simulink model "write_data_2018a"  (R2018a)
settings: Solver=FixedStepAuto  StartTime=0.0  StopTime=0.0001  RelTol=1e-3
values from neighbouring files (symbols this model uses):
  transfer_array = zeros(1,30)    [final_test.m]    (also in main_file.m = calc_corr_arr(transfer_array, v_m))
libraries: TcAdsLib x3
settings Model: Creator=chijiang  LastModifiedBy=chduan
settings OptimizationCC: LocalBlockOutputs=off
settings SFSimCC: SimUseLocalCustomCode=on
settings RTWCC: SystemTargetFile=TwinCAT.tlc  MakeCommand=make_tct  TemplateMakefile=tct_msbuild.tmf  Description=TwinCAT Target  GenerateReport=on  RTWUseLocalCustomCode=on  TargetLang=C++
settings STFCustomTargetCC: TargetLangStandard=C++03 (ISO)  CompOptLevelCompliant=on  MATLABClassNameForMDSCustomization=Simulink.SoftwareTarget.TargetSpecificTriggerConfigurationBase  SystemTargetFile=TwinCAT.tlc

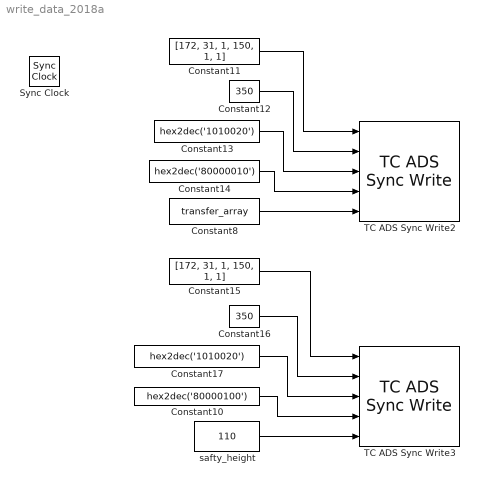
== system write_data_2018a ==
  Constant10 : Constant  Value=hex2dec('80000100')  OutDataTypeStr=uint32
  Constant11 : Constant  Value=[172, 31, 1, 150, 1, 1]  OutDataTypeStr=uint8
  Constant12 : Constant  Value=350  OutDataTypeStr=uint16
  Constant13 : Constant  Value=hex2dec('1010020')  OutDataTypeStr=uint32
  Constant14 : Constant  Value=hex2dec('80000010')  OutDataTypeStr=uint32
  Constant15 : Constant  Value=[172, 31, 1, 150, 1, 1]  OutDataTypeStr=uint8
  Constant16 : Constant  Value=350  OutDataTypeStr=uint16
  Constant17 : Constant  Value=hex2dec('1010020')  OutDataTypeStr=uint32
  Constant8 : Constant  Value=transfer_array
  Sync Clock : TcAdsLib/Utilities/Sync Clock  OutputPortSelect=None  InputPortSelect=None
      settings: SourceProductName=Beckhoff TwinCAT ADS Interface
  TC ADS Sync Write2 : TcAdsLib/Synchronous/TC ADS Sync Write  SampleTime=-1  AbortSimulationOnAdsError=off  WriteDataType=double  WriteDataDim=30  WriteDataColToRowMajor=on  AdsTimeout=1  DirectFeedThrough=off  CreateSignalLabels=on  CodeGenConnectType=DataArea (OutputSrc)
      settings: SourceProductName=Beckhoff TwinCAT ADS Interface
  TC ADS Sync Write3 : TcAdsLib/Synchronous/TC ADS Sync Write  SampleTime=-1  AbortSimulationOnAdsError=off  WriteDataType=double  WriteDataDim=1  WriteDataColToRowMajor=on  AdsTimeout=1  DirectFeedThrough=off  CreateSignalLabels=on  CodeGenConnectType=DataArea (OutputSrc)
      settings: SourceProductName=Beckhoff TwinCAT ADS Interface
  safty_height : Constant  Value=110
  wires:
  Constant10/1 -> TC ADS Sync Write3/4
  Constant17/1 -> TC ADS Sync Write3/3
  Constant11/1 -> TC ADS Sync Write2/1
  Constant8/1 -> TC ADS Sync Write2/5
  Constant14/1 -> TC ADS Sync Write2/4
  Constant16/1 -> TC ADS Sync Write3/2
  Constant15/1 -> TC ADS Sync Write3/1
  safty_height/1 -> TC ADS Sync Write3/5
  Constant12/1 -> TC ADS Sync Write2/2
  Constant13/1 -> TC ADS Sync Write2/3
